simulink model "Navrh_ref_modelu_S_2"  (R2023b)
settings: Solver=ode45  StartTime=0.0  StopTime=15  RelTol=1e-3  EnableMultiTasking=on
model workspace (MAT data in the model file):
  Am = [-1.66666666667  0  0; 0  0  1; 0  -0.444444444444  -1.33333333333]
  Bm = [1.66666666667  0; 0  0; 0  0.444444444444]
  T1 = 0.6
  T2 = 1.5
settings Model: Creator=PF  LastModifiedBy=ivanz
settings SolverCC: AlgebraicLoopSolver=TrustRegion
settings DataIOCC: LimitDataPoints=on  SaveFormat=Array  SignalLoggingSaveFormat=ModelDataLogs  ReturnWorkspaceOutputs=off  SignalLoggingName=sigsOut
settings OptimizationCC: InitFltsAndDblsToZero=on  LifeSpan=inf
settings DebuggingCC: SaveWithParameterizedLinksMsg=none  UnderspecifiedInitializationDetection=Classic  MergeDetectMultiDrivingBlocksExec=none  SignalResolutionControl=TryResolveAllWithWarning  MultiTaskDSMMsg=warning  MultiTaskCondExecSysMsg=none  FcnCallInpInsideContextMsg=warning  UnconnectedInputMsg=warning  UnconnectedOutputMsg=warning  UnconnectedLineMsg=warning  SFUnexpectedBacktrackingDiag=warning  SFNoUnconditionalDefaultTransitionDiag=warning  SFExecutionAtInitializationDiag=none  ArithmeticOperatorsInVariantConditions=warning
settings HardwareCC: ProdBitPerPointer=32  ProdBitPerSizeT=32  ProdBitPerPtrDiffT=32  ProdLargestAtomicFloat=None  ProdIntDivRoundTo=Undefined  ProdEndianess=Unspecified  ProdWordSize=32  ProdHWDeviceType=32-bit Generic  TargetUnknown=on
settings ModelReferenceCC: EnableRefExpFcnMdlSchedulingChecks=on  PropagateSignalLabelsOutOfModel=off
settings RTWCC: DLArmComputeVersion=19.05
settings CodeAppCC: StateflowObjectComments=on
settings GRTTargetCC: TargetFcnLib=ansi_tfl_tmw.mat  TargetLangStandard=C89/C90 (ANSI)  CombineOutputUpdateFcns=off  GRTInterface=on
settings ConfigComp: CovMetricSettings=dw  CovSaveCumulativeToWorkspaceVar=on  CovSaveSingleToWorkspaceVar=on

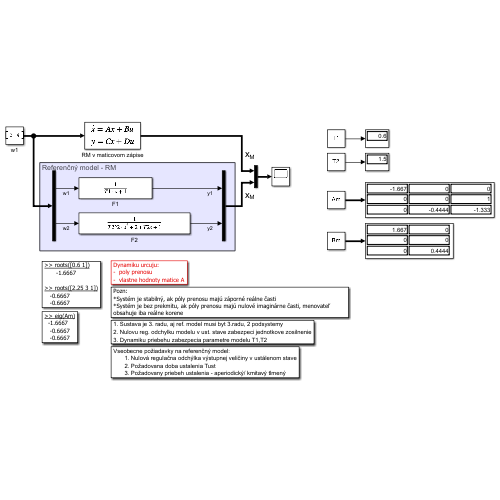
[thumbnail: Simulink's stored preview of the top-level diagram]
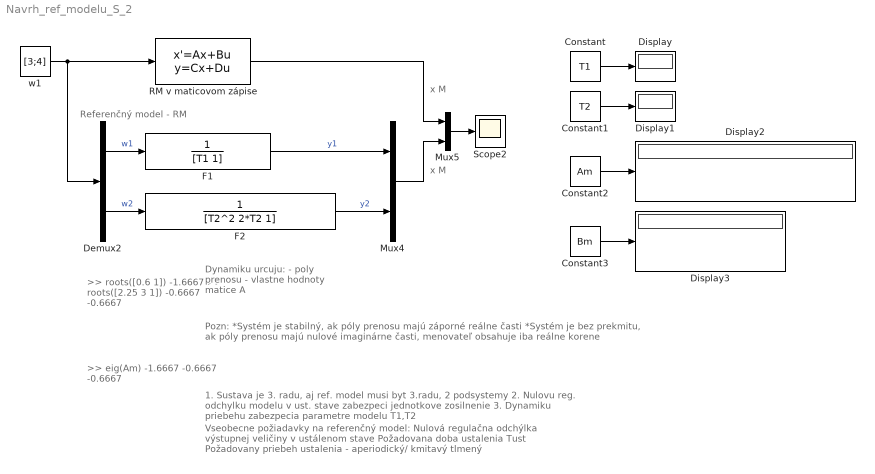
== system Navrh_ref_modelu_S_2 ==
  note: Referenčný model - RM
  note: >> eig(Am)
      | -1.6667
      | -0.6667
      | -0.6667
  note: >> roots([0.6 1])
      | -1.6667
      |
      | >> roots([2.25 3 1])
      | -0.6667
      | -0.6667
  note: Pozn:
      | *Systém je stabilný, ak póly prenosu majú záporné reálne časti
      | *Systém je bez prekmitu, ak póly prenosu majú nulové imaginárne časti, menovateľ obsahuje iba reálne korene
  note: Dynamiku urcuju:
      | - poly prenosu
      | - vlastne hodnoty matice A
  note: x M
  note: x M
  note: 1. Sustava je 3. radu, aj ref. model musi byt 3.radu, 2 podsystemy
      | 2. Nulovu reg. odchylku modelu v ust. stave zabezpeci jednotkove zosilnenie
      | 3. Dynamiku priebehu zabezpecia parametre modelu T1,T2
  note: Vseobecne požiadavky na referenčný model:
      | Nulová regulačna odchýlka výstupnej veličiny v ustálenom stave
      | Požadovana doba ustalenia Tust
      | Požadovany priebeh ustalenia - aperiodický/ kmitavý tlmený
  Constant : Constant  Value=T1
  Constant1 : Constant  Value=T2
  Constant2 : Constant  Value=Am
  Constant3 : Constant  Value=Bm
  Demux2 : Demux  Outputs=2
  Display{,1..3} (4 alike) : Display
  F1 : TransferFcn  Denominator=[T1 1]
  F2 : TransferFcn  Denominator=[T2^2 2*T2 1]
  Mux4 : Mux  Inputs=2
  Mux5 : Mux  Inputs=2
  RM v maticovom zápise : StateSpace  A=[-1/T1 0 0; 0 0 1; 0 -1/T2^2 -2/T2]  B=[1/T1 0; 0 0; 0 1/T2^2]  C=[1 0 0;0 1 0; 0 0 1]  D=[0 0;0 0;0 0]  InitialCondition=0
  Scope2 : Scope
  w1 : Constant  Value=[3;4]
  wires:
  Mux5/1 -> Scope2/1
  Mux4/1 -> Mux5/2
  RM v maticovom zápise/1 -> Mux5/1
  F1/1 -> Mux4/1  "y1"
  Demux2/2 -> F2/1  "w2"
  w1/1 -> Demux2/1, RM v maticovom zápise/1
  Demux2/1 -> F1/1  "w1"
  F2/1 -> Mux4/2  "y2"
  Constant1/1 -> Display1/1
  Constant/1 -> Display/1
  Constant2/1 -> Display2/1
  Constant3/1 -> Display3/1
